simulink model "totalsystem_final_working"  (R2015b)
settings: Solver=ode45  StartTime=0.0  StopTime=50.0  RelTol=1e-5
libraries: simulink x2
settings Model: Creator=Labo  LastModifiedBy=thoma
settings DataIOCC: SaveFormat=Array  SignalLoggingSaveFormat=ModelDataLogs
settings DebuggingCC: UnderspecifiedInitializationDetection=Classic  MergeDetectMultiDrivingBlocksExec=none  SolverPrmCheckMsg=warning  MultiTaskDSMMsg=warning  MultiTaskCondExecSysMsg=none  StateNameClashWarn=warning
settings HardwareCC: ProdBitPerPointer=32  ProdLargestAtomicFloat=None  ProdIntDivRoundTo=Undefined  ProdEndianess=Unspecified  ProdWordSize=32  ProdHWDeviceType=32-bit Generic
settings GRTTargetCC: GeneratePreprocessorConditionals=Disable all
settings ConfigComp: CovModelRefEnable=Off

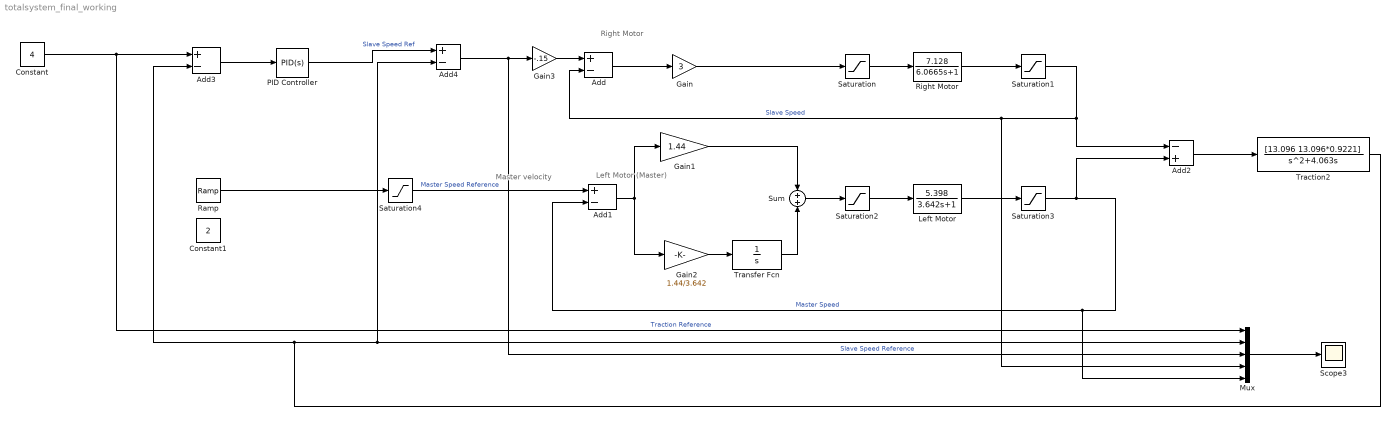
== system totalsystem_final_working ==
  note: Master velocity
  note: Left Motor (Master)
  note: Right Motor
  Add{,1,3..4} (4 alike) : Sum  Inputs=+-
  Add2 : Sum  Inputs=-+
  Constant : Constant  Value=4
  Constant1 : Constant  Value=2
  Gain : Gain  Gain=3
  Gain1 : Gain  Gain=1.44
  Gain2 : Gain  Gain=1.44/3.642
  Gain3 : Gain  Gain=-.15
  "Left Motor " : TransferFcn  Numerator=[5.398]  Denominator=[3.642 1]  ContinuousStateAttributes='v'
  Mux : Mux  Inputs=5
  PID Controller : simulink/Continuous/PID Controller  Controller=PID  TimeDomain=Continuous-time  SampleTime=-1  IntegratorMethod=Forward Euler  FilterMethod=Forward Euler  Form=Parallel  UseFilter=on  ControllerParametersSource=internal  P=4  I=2.06*4  D=0  N=100  InitialConditionSource=internal  InitialConditionForIntegrator=0  InitialConditionForFilter=0  ExternalReset=none  LimitOutput=off  UpperSaturationLimit=inf  LowerSaturationLimit=-inf  LinearizeAsGain=on  AntiWindupMode=none  Kb=1  TrackingMode=off  Kt=1  PParamMin=[]  PParamMax=[]  IParamMin=[]  IParamMax=[]  DParamMin=[]  DParamMax=[]  NParamMin=[]  NParamMax=[]  KbParamMin=[]  KbParamMax=[]  KtParamMin=[]  KtParamMax=[]  POutMin=[]  POutMax=[]  IOutMin=[]  IOutMax=[]  DOutMin=[]  DOutMax=[]  NOutMin=[]  NOutMax=[]  KbOutMin=[]  KbOutMax=[]  KtOutMin=[]  KtOutMax=[]  IntegratorOutMin=[]  IntegratorOutMax=[]  FilterOutMin=[]  FilterOutMax=[]  SumOutMin=[]  SumOutMax=[]  SumI1OutMin=[]  SumI1OutMax=[]  SumI2OutMin=[]  SumI2OutMax=[]  SumI3OutMin=[]  SumI3OutMax=[]  SumDOutMin=[]  SumDOutMax=[]  SaturationOutMin=[]  SaturationOutMax=[]  IntegratorContinuousStateAttributes=''  IntegratorStateMustResolveToSignalObject=off  IntegratorRTWStateStorageClass=Auto  FilterContinuousStateAttributes=''  FilterStateMustResolveToSignalObject=off  FilterRTWStateStorageClass=Auto  DifferentiatorICPrevScaledInput=0  DifferentiatorOutMin=[]  DifferentiatorOutMax=[]
  Ramp : simulink/Sources/Ramp  slope=2/8  start=0  X0=0
  "Right Motor " : TransferFcn  Numerator=[7.128]  Denominator=[6.0665 1]  ContinuousStateAttributes='v'
  Saturation : Saturate  UpperLimit=7.3  LowerLimit=-17.3
  Saturation1 : Saturate  UpperLimit=10-2.79  LowerLimit=-10-2.79
  Saturation2 : Saturate  UpperLimit=7.3  LowerLimit=-17.3
  Saturation3 : Saturate  UpperLimit=10-8.623  LowerLimit=-10-8.623
  Saturation4 : Saturate  UpperLimit=2  LowerLimit=0
  Scope3 : Scope
  Sum : Sum  Inputs=+|+
  Traction2 : TransferFcn  Numerator=[13.096 13.096*0.9221]  Denominator=[1 4.063 0]
  Transfer Fcn : TransferFcn  Denominator=[1 0]
  wires:
  Add/1 -> Gain/1
  "Right Motor "/1 -> Saturation1/1
  Saturation1/1 -> Add2/1, Mux/4, Add/2  "Slave Speed"
  Saturation/1 -> "Right Motor "/1
  Add1/1 -> Gain2/1, Gain1/1
  "Left Motor "/1 -> Saturation3/1
  Saturation3/1 -> Mux/5, Add1/2, Add2/2  "Master Speed"
  Saturation2/1 -> "Left Motor "/1
  Sum/1 -> Saturation2/1
  Traction2/1 -> Add4/2, Mux/2, Add3/2
  Constant/1 -> Add3/1, Mux/1  "Traction Reference"
  Saturation4/1 -> Add1/1  "Master Speed Reference"
  Mux/1 -> Scope3/1
  Add2/1 -> Traction2/1
  Gain2/1 -> Transfer Fcn/1
  Transfer Fcn/1 -> Sum/2
  Gain1/1 -> Sum/1
  Add3/1 -> PID Controller/1
  Gain/1 -> Saturation/1
  Add4/1 -> Gain3/1, Mux/3  "Slave Speed Reference"
  Ramp/1 -> Saturation4/1
  Gain3/1 -> Add/1
  PID Controller/1 -> Add4/1  "Slave Speed Ref"
